simulink model "PACEMAKER"  (R2022b)
settings: Solver=FixedStepAuto  StartTime=0.0  StopTime=10.0  FixedStep=1e-3  RelTol=1e-3  EnableMultiTasking=on
libraries: frdmk64flib x2
settings Model: ExtModeTrigDuration=5  Creator=mutha  LastModifiedBy=jathe
settings SolverCC: AlgebraicLoopSolver=TrustRegion
settings OptimizationCC: EnhancedBackFolding=on  PassReuseOutputArgsAs=Individual arguments  ZeroExternalMemoryAtStartup=off  ZeroInternalMemoryAtStartup=off  MaxStackSize=64  OptimizeBlockOrder=speed  DifferentSizesBufferReuse=on  OptimizationCustomize=off  EfficientTunableParamExpr=on
settings DebuggingCC: ParameterTunabilityLossMsg=error  UnconnectedInputMsg=warning  UnconnectedOutputMsg=warning  UnconnectedLineMsg=warning  SFMachineParentedDataDiag=warning
settings HardwareCC: ProdBitPerPointer=32  ProdBitPerSizeT=32  ProdBitPerPtrDiffT=32  ProdLargestAtomicInteger=Long  ProdLargestAtomicFloat=Double  ProdWordSize=32  ProdHWDeviceType=ARM Compatible->ARM Cortex
settings ModelReferenceCC: EnableRefExpFcnMdlSchedulingChecks=on
settings SFSimCC: MATLABDynamicMemAlloc=off
settings RTWCC: Description=Embedded Coder  SystemTargetFile=ert.tlc  HardwareBoard=NXP FRDM-K64F  TLCOptions="-aInlineSetEventsForThisBaseRateFcn=TLC_FALSE -aSuppressMultiTaskScheduler=TLC_FALSE  -aRateBasedStepFcn=0"  TemplateMakefile=ert_default_tmf  Toolchain=GNU Tools for ARM Embedded Processors  DLArmComputeVersion=19.05
settings CodeAppCC: ForceParamTrailComments=on  IgnoreCustomStorageClasses=off  OperatorAnnotations=on  SimulinkDataObjDesc=on  SFDataObjDesc=on  InsertBlockDesc=on
settings ERTTargetCC: ExtModeTransport=4  ExtModeMexFile=sendToCommService

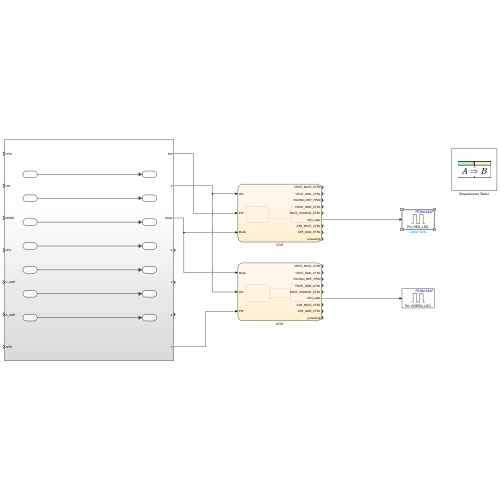
[thumbnail: Simulink's stored preview of the top-level diagram]
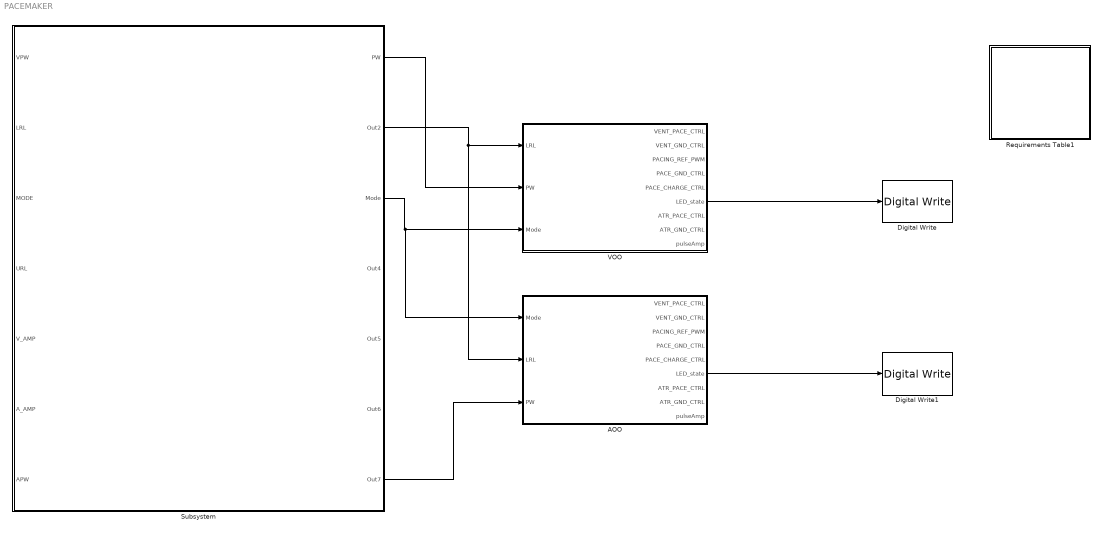
== system PACEMAKER ==
  AOO : Stateflow chart  TreatAsAtomicUnit=on
      settings: PortSchema="{\"entries\":[{\"content\":{\"sides\":[{\"content\":{\"connectorIds\":[\"In3\",\"In1\",\"In2\"]},\"type\":\"ConnectorPlacement.EquallySpacedRectSide\",\"uuid\":\"4a9106b9-4977-4ad7-a664-79baeb9488d7\"},{\"content\":{\"connectorIds\":[\"Out1\",\"Out2\",\"Out3\",\"Out4\",\"Out5\",\"Out6\",\"Out7\",\"Out8\",\"Out9\"],\"side\":\"RIGHT\"},\"type\":\"ConnectorPlacement.EquallySpacedRectSide\",\"uuid\":\"b9887666-f10a-4603-9f8e-4ad73175cafe\"},{\"content\":{\"connectorIds\":[],\"side\":\"TOP\"},\"type\":\"ConnectorPlacement.EquallySpacedRectSide\",\"uuid\":\"1850edd3-c966-4e07-b98a-67abbc5f02e7\"}]},\"type\":\"ConnectorPlacement.EquallySpacedConnector\",\"uuid\":\"2b9e48c6-c28a-4e83-8c86-f722f9137b29\"}],\"packageUris\":[\"http://schema.mathworks.com/mf0/Connector/R2020b\"],\"version\":\"1.0\"}"
  Digital Write : frdmk64flib/Digital Write  Whichpin=RED_LED
  Digital Write1 : frdmk64flib/Digital Write  Whichpin=GREEN_LED
  Requirements Table1 : Requirements Table  TreatAsAtomicUnit=on
  Subsystem : Subsystem
  VOO : Stateflow chart  TreatAsAtomicUnit=on
  wires:
  VOO/6(LED_state) -> Digital Write/1
  AOO/6(LED_state) -> Digital Write1/1
  Subsystem/2(Out2) -> AOO/1(LRL), VOO/1(LRL)
  Subsystem/1(PW) -> VOO/2(PW)
  Subsystem/7(Out7) -> AOO/2(PW)
  Subsystem/3(Mode) -> AOO/3(Mode), VOO/3(Mode)

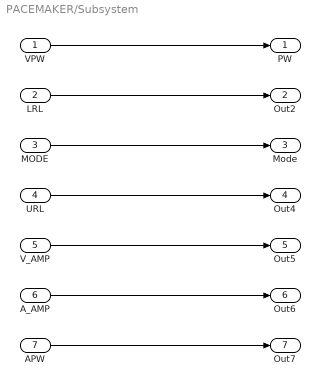
== system PACEMAKER/Subsystem ==
  VPW : Inport
  LRL : Inport  Port=2
  MODE : Inport  Port=3
  URL : Inport  Port=4
  V_AMP : Inport  Port=5
  A_AMP : Inport  Port=6
  APW : Inport  Port=7
  PW : Outport
  Out2 : Outport  Port=2
  Mode : Outport  Port=3
  Out4 : Outport  Port=4
  Out5 : Outport  Port=5
  Out6 : Outport  Port=6
  Out7 : Outport  Port=7
  wires:
  VPW/1 -> PW/1
  LRL/1 -> Out2/1
  MODE/1 -> Mode/1
  URL/1 -> Out4/1
  V_AMP/1 -> Out5/1
  A_AMP/1 -> Out6/1
  APW/1 -> Out7/1

== stateflow chart PACEMAKER/Requirements Table1 ==
  (default) -> (junction 1073742112)
  (junction 1073742112) -> (junction 1073742113) : {
      | % SF_REQ_REV_07
      | }
  (junction 1073742113) -> (junction 1073742115) : {
      | % HEADER_ASSIGNMENTS
      |
      | }
  (junction 1073742115) -> (junction 1073742117) : {
      | % START_A_4
      | }
  (junction 1073742117) -> (junction 1073742119) : {
      | }
  (junction 1073742119) -> (junction 1073742121)
  (junction 1073742121) -> (junction 1073742123) : {
      | }
  (junction 1073742123) -> (junction 1073742125) : {
      | % END_A_4
      | }
  (junction 1073742125) -> (junction 1073742127) : {
      | % START_R_1
      | }
  (junction 1073742127) -> (junction 1073742129) : {
      | }
  (junction 1073742129) -> (junction 1073742131)
  (junction 1073742131) -> (junction 1073742133) [order 1] : [duration((((Mode) == (1))) && (((LED) == (LED_off)))) >= PW]
  (junction 1073742131) -> (junction 1073742157) [order 2]
  (junction 1073742133) -> (junction 1073742135) : {
      | reqtable_postcondition((((High Conditions) == (VENT HIGH))), 'R:1');
      | LED_on
      |
      | }
  (junction 1073742135) -> (junction 1073742137) : {
      | }
  (junction 1073742137) -> (junction 1073742139) : {
      | % START_R_7
      | }
  (junction 1073742139) -> (junction 1073742141) : {
      | }
  (junction 1073742141) -> (junction 1073742143)
  (junction 1073742143) -> (junction 1073742145) [order 1] : [duration((((Mode) == (1))) && (((LED) == (LED_on)))) >= (60/LRL) - PW]
  (junction 1073742143) -> (junction 1073742151) [order 2]
  (junction 1073742145) -> (junction 1073742147) : {
      | reqtable_postcondition((((High Conditions) == (VENT LOW ))), 'R:1.1');
      | LED_off
      |
      | }
  (junction 1073742147) -> (junction 1073742149) : {
      | }
  (junction 1073742149) -> (junction 1073742151)
  (junction 1073742151) -> (junction 1073742153)
  (junction 1073742153) -> (junction 1073742155) : {
      | % END_R_7
      | }
  (junction 1073742155) -> (junction 1073742157)
  (junction 1073742157) -> (junction 1073742159)
  (junction 1073742159) -> (junction 1073742161) : {
      | % END_R_1
      | }

== stateflow chart PACEMAKER/AOO ==
  state LED_off %State 1(VOO)
    %Charging C22
    Mode = 2;
    PACING_REF_PWM = (pulseAmp / 5);
    PACE_CHARGE_CTRL = true;
    VENT_PACE_CTRL = false;
    ATR_PACE_CTRL = false;
    %Discharging C21
    PACE_GND_CTRL = true;
    VENT_GND_CTRL = false;
    ATR_GND_CTRL = true;
    %LED STATE
    LED_state = false;
  state LED_on%State2(VOO)
    %Discharging C22
    PACE_CHARGE_CTRL = false;
    PACE_GND_CTRL = true;
    VENT_PACE_CTRL = false;
    ATR_PACE_CTRL = true;
    VENT_GND_CTRL = true; %not sure
    ATR_GND_CTRL = false;
    %LED STATE
    LED_state = true;
  (default) -> LED_off %State 1(VOO)
  LED_off %State 1(VOO) -> LED_on%State2(VOO) : after (PW,msec)
  LED_on%State2(VOO) -> LED_off %State 1(VOO) : after ((60000/LRL) - PW, msec)
  data: VENT_PACE_CTRL output boolean; VENT_GND_CTRL output boolean; PACING_REF_PWM output int8; PACE_GND_CTRL output boolean; PACE_CHARGE_CTRL output boolean; LED_state output boolean; ATR_PACE_CTRL output boolean; ATR_GND_CTRL output boolean; pulseAmp output int8; LRL input int8; PW input int8; Mode input int8

== stateflow chart PACEMAKER/VOO ==
  state LED_off %State 1(VOO)
    Mode = 1;
    %Charging C22
    PACING_REF_PWM = (pulseAmp / 5);
    PACE_CHARGE_CTRL = true;
    VENT_PACE_CTRL = false;
    ATR_PACE_CTRL = false;
    %Discharging C21
    PACE_GND_CTRL = true;
    VENT_GND_CTRL = true;
    ATR_GND_CTRL = false;
    %LED STATE
    LED_state = false;
  state LED_on%State2(VOO)
    Mode = 1;
    %Discharging C22
    PACE_CHARGE_CTRL = false;
    PACE_GND_CTRL = true;
    VENT_PACE_CTRL = true;
    ATR_PACE_CTRL = false;
    VENT_GND_CTRL = false;
    ATR_GND_CTRL = true; %not sure
    %LED STATE
    LED_state = true;
  (default) -> LED_off %State 1(VOO)
  LED_off %State 1(VOO) -> LED_on%State2(VOO) : after (PW,msec)
  LED_on%State2(VOO) -> LED_off %State 1(VOO) : after ((60000/LRL) - PW, msec)
  data: VENT_PACE_CTRL output boolean; VENT_GND_CTRL output boolean; PACING_REF_PWM output int8; PACE_GND_CTRL output boolean; PACE_CHARGE_CTRL output boolean; LED_state output boolean; ATR_PACE_CTRL output boolean; ATR_GND_CTRL output boolean; pulseAmp output int8; LRL input int8; PW input int8; Mode input
